simulink model "sf_1_simple_model"  (R2022b)
settings: Solver=VariableStepAuto  StartTime=0.0  StopTime=inf  RelTol=1e-3
settings Model: Creator=user  LastModifiedBy=user

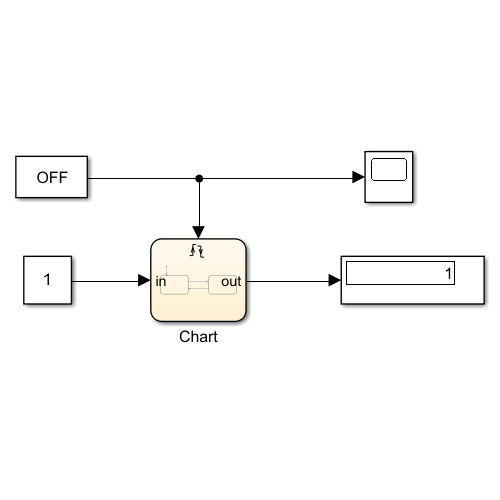
[thumbnail: Simulink's stored preview of the top-level diagram]
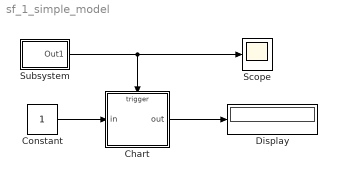
== system sf_1_simple_model ==
  Chart : Stateflow chart  TreatAsAtomicUnit=on
  Constant : Constant
  Display : Display
  Scope : Scope
  Subsystem : Subsystem  StartFcn=|  mask{str=OFF}
      | set_param(gcb, 'str', 'OFF');
      | set_param([gcb,'/C'], 'Value', '0');
      mask prompts: str "Display Name :"
      settings: OpenFcn=|
      | old_val = get_param([gcb, '/C'], 'Value');
      | 
      | switch old_val
      |  case '0'
      |   set_param(gcb, 'str', 'ON');
      |   set_param([gcb, '/C'], 'Value', '1');
      |  case '1'
      |   set_param(gcb, 'str', 'OFF');
      |   set_param([gcb,'/C'], 'Value', '0');
      |  otherwise
      |   set_param(gcb, 'str', 'OFF');
      |   set_param([gcb,'/C'], 'Value', '0');
      | end
      mask DialogControl ParameterGroupVar Prompt: 파라미터
      mask Display:
      | blk_name = get_param(gcb, 'str');
      | disp(blk_name);
  wires:
  Constant/1 -> Chart/1(in)
  Chart/1(out) -> Display/1
  Subsystem/1(Out1) -> Scope/1, Chart/Trigger

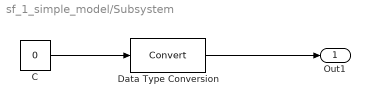
== system sf_1_simple_model/Subsystem ==
  C : Constant  Value=0
  Data Type Conversion : DataTypeConversion  SaturateOnIntegerOverflow=off  RndMeth=Floor
  Out1 : Outport
  wires:
  C/1 -> Data Type Conversion/1
  Data Type Conversion/1 -> Out1/1

== stateflow chart sf_1_simple_model/Chart ==
  settings: executeAtInitialization=1
  state POS
    entry : out = in;
  state NEG
    entry : out = -in;
  (default) -> POS
  POS -> NEG : E
  NEG -> POS : E
  data: in input; out output
  events: E input EITHER_EDGE_EVENT
